simulink model "e03_MtrCtrl_MtrCtrl"  (R2024a)
settings: Solver=FixedStepDiscrete  StartTime=0.0  StopTime=1  FixedStep=mSim.dTime  MaxStep=Define.sModelSampleTime  RelTol=7.1420e-05
undefined symbols (not defined in the file): CnstCnst, CnstMde, CnstNr, E03CCTRL, E03INIT, E03LIM, E03MCMV, sTempGain
libraries: Lib_LPF x2
(part 2 of 3)

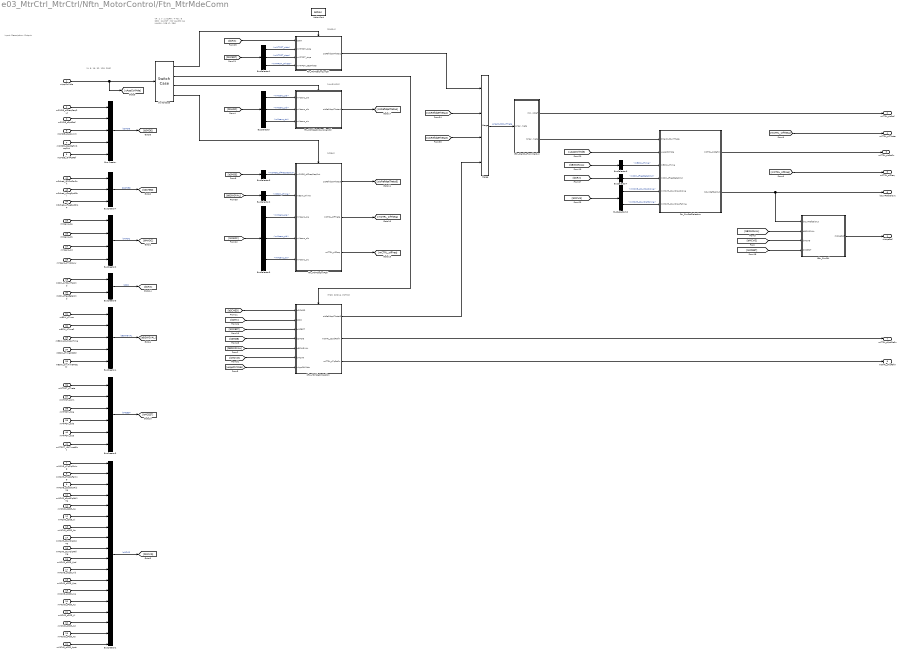
== system e03_MtrCtrl_MtrCtrl/Nftn_MotorControl/Ftn_MtrMdeComn ==
  note: [4, 8, 16, 32, 128, 256]
  note: Input:
      | Description:
      | Output:
  note: VF : 1
      | V : 2
      | CURR : 4
      | TQ : 8
      | SPD : 16
      | PST : 32
      | VALIGN: 64
      | IALIGN : 128
      | IF : 256
  note: [IF256]
  note: [CURR4]
  note: [IALIGN128]
  note: [TQ8, SPD16, PST32]
  uAppCtrlMde : Inport  Description=■ 설명: 모터 구동 제어 모드  OutMin=0  OutMax=32
      settings: AttributesFormatString=%<Description>
  mSMDE_sIfFreqSeqOut : Inport  Description=■ 설명: IF Control Frequency out  Port=2  OutMin=0  OutMax=54
      settings: AttributesFormatString=%<Description>
  mSMDE_sSpdRef : Inport  Description=■ 설명: Speed Reference  Port=3  OutMin=0  OutMax=11000
      settings: AttributesFormatString=%<Description>
  mSMDE_sSpdRefInSeqOut : Inport  Description=■ 설명: Speed Reference Slop Out  Port=4  OutMin=0  OutMax=11000
      settings: AttributesFormatString=%<Description>
  mSMDE_i64PstRef : Inport  Description=■ 설명: Position Reference  Port=5
      settings: AttributesFormatString=%<Description>
  mSMDE_sSpdLimit : Inport  Description='■ 설명: 속도 제한값  Port=6
      settings: AttributesFormatString=%<Description>
  mMCVG_sTqSlpRising : Inport  Description=■ 설명: 토크 제어 지령 가속 기울기  Port=7
      settings: AttributesFormatString=%<Description>
  mMCVG_sTqSlpFalling : Inport  Description=■ 설명: 토크 제어 지령 감속 기울기  Port=8
      settings: AttributesFormatString=%<Description>
  mMCVG_sSpdSlpRising : Inport  Description=■ 설명: Speed Slop Rising Gain  Port=9  OutMin=0  OutMax=3000
      settings: AttributesFormatString=%<Description>
  mMCVG_sSpdSlpFalling : Inport  Description=■ 설명: Speed Slop Falling Gain  Port=10  OutMin=0  OutMax=3000
      settings: AttributesFormatString=%<Description>
  mMCVG_sSCG_Kp : Inport  Description=■ 설명: Speed Gain Kp Gain  Port=11  OutMin=0  OutMax=10
      settings: AttributesFormatString=%<Description>
  mMCVG_sSCG_Ki : Inport  Description=■ 설명: Speed Gain Ki Gain  Port=12  OutMin=0  OutMax=10
      settings: AttributesFormatString=%<Description>
  mMCVG_sSCG_Ka : Inport  Description=■ 설명: Speed Gain Ka Gain  Port=13  OutMin=0  OutMax=100
      settings: AttributesFormatString=%<Description>
  mMCVG_sCurrSlpRising : Inport  Description=■ 설명: Current Rising Slop Gain  Port=14  OutMin=0  OutMax=5000
      settings: AttributesFormatString=%<Description>
  mMCVG_sCurrSlpFalling : Inport  Description=■ 설명: Current Falling Slop Gain  Port=15  OutMin=0  OutMax=5000
      settings: AttributesFormatString=%<Description>
  mMCVG_sCCG_Kpd : Inport  Description=■ d축 전류 제어 게인 Kp  Port=16  OutMin=0  OutMax=100
      settings: AttributesFormatString=%<Description>
  mMCVG_sCCG_Kid : Inport  Description=■ d축 전류 제어 게인 Ki  Port=17  OutMin=0  OutMax=100
      settings: AttributesFormatString=%<Description>
  mMCVG_sCCG_Kpq : Inport  Description=■ 설명: Current Gain Kp Gain  Port=18  OutMin=0  OutMax=100
      settings: AttributesFormatString=%<Description>
  mMCVG_sCCG_Kiq : Inport  Description=■ 설명: Current Gain Ki Gain  Port=19  OutMin=0  OutMax=100
      settings: AttributesFormatString=%<Description>
  mMCVG_sPCG_Kp : Inport  Description=■ 설명: 위치 제어 게인 Kp  Port=20
      settings: AttributesFormatString=%<Description>
  mMCVG_sPCG_Ki : Inport  Description=■ 설명: 위치 제어 게인 Ki  Port=21
      settings: AttributesFormatString=%<Description>
  mMCVG_sPCG_Kd : Inport  Description=■ 설명: 위치 제어 게인 Kd  Port=22
      settings: AttributesFormatString=%<Description>
  mMCVG_sPCG_Ka : Inport  Description=■ 설명: 위치 제어 게인 Ka  Port=23
      settings: AttributesFormatString=%<Description>
  mMCVG_sPCG_Apst : Inport  Description=■ 설명: 가속도 게인  Port=24
      settings: AttributesFormatString=%<Description>
  mMsens_sIa : Inport  Description=■ 설명: 모터 A상 전류  Port=25  OutMin=-162.6  OutMax=162.6
      settings: AttributesFormatString=%<Description>
  mMsens_sIb : Inport  Description=■ 설명: 모터 B상 전류  Port=26  OutMin=-162.6  OutMax=162.6
      settings: AttributesFormatString=%<Description>
  mMsens_sIc : Inport  Description=■ 설명: 모터 C상 전류  Port=27  OutMin=-325.2  OutMax=325.2
      settings: AttributesFormatString=%<Description>
  mMsens_sHVdcLow : Inport  Description=■ 설명: HVdc 전압  Port=28  OutMin=0  OutMax=1000
      settings: AttributesFormatString=%<Description>
  mCRX_sVltCurrTqCmd : Inport  Description=■ 설명: uVltCurrTqCmd(Voltage / Current / Torque Reference)  Port=29  OutMin=-398.3  OutMax=398.3
      settings: AttributesFormatString=%<Description>
  mCRX_sFreqBetaCmd : Inport  Description=■ 설명: uFreqBetaCmd(Frequency / Beta Reference)  Port=30  OutMin=0  OutMax=409.5
      settings: AttributesFormatString=%<Description>
  mBSW_sTime : Inport  Description=■ 설명: 주기, sTime (1/14kH)  Port=31  OutMin=0  OutMax=0.0000714286
      settings: AttributesFormatString=%<Description>
  mBSW_sTime2 : Inport  Description=■ 설명: sTime * 2  Port=32  OutMin=0  OutMax=0.000142857
      settings: AttributesFormatString=%<Description>
  mBSW_sOutloopTime : Inport  Description=■ 설명: sTime * 10  Port=33  OutMin=0  OutMax=0.000714286
      settings: AttributesFormatString=%<Description>
  mBSW_sTimePstCtrl : Inport  Description=■ 설명: Main Task 30배 주기  Port=34
      settings: AttributesFormatString=%<Description>
  mBSW_sInvTimePstCtrl : Inport  Description=■ 설명: mBSW_sTimePstCtrl의 역수  Port=35
      settings: AttributesFormatString=%<Description>
  mMTPST_sTheta : Inport  Description=■ 설명: Rotor Position  Port=36  OutMin=0  OutMax=6.2832
      settings: AttributesFormatString=%<Description>
  mMTPST_sWm : Inport  Description=■ 설명: 기계 각속도 (Wm = 12000 * 2pi/60)  Port=37  OutMin=0  OutMax=1256.63706
      settings: AttributesFormatString=%<Description>
  mMTPST_sWe : Inport  Description=■ 설명: 전기 각속도 (We = Wm * Poles)  Port=38  OutMin=0  OutMax=5026.55
      settings: AttributesFormatString=%<Description>
  mMTPST_sIde : Inport  Description=■ 설명: sIde  Port=39  OutMin=-398.3  OutMax=398.3
      settings: AttributesFormatString=%<Description>
  mMTPST_sIqe : Inport  Description=■ 설명: sIqe  Port=40  OutMin=-398.3  OutMax=398.3
      settings: AttributesFormatString=%<Description>
  mMTPST_i64TurretPst : Inport  Description=■ 설명: Turret Position  Port=41
      settings: AttributesFormatString=%<Description>
  mSched_i32CntForSch : Inport  Description=■ 설명: 메인 스케쥴 카운터  Port=42
      settings: AttributesFormatString=%<Description>
  mSched_uFlagSpdCtrl : Inport  Description=■ 설명: Speed Control 스케쥴 카운터  Port=43  OutMin=0  OutMax=1
      settings: AttributesFormatString=%<Description>
  mSched_uFlagSpdSlop : Inport  Description=■ 설명: 속도 지령 Slop 스케쥴 카운터  Port=44  OutMin=0  OutMax=1
      settings: AttributesFormatString=%<Description>
  ActionPort : ActionPort  ActionPortLabel=case [ 4 8 16 32 128 256 ]:
  Bus Creator : BusCreator  Inputs=5
  BusCreator1 : BusCreator  Inputs=18
  BusCreator2 : BusCreator  Inputs=4
  BusCreator3 : BusCreator  Inputs=2
  BusCreator4 : BusCreator  Inputs=5
  BusCreator5 : BusCreator  Inputs=6
  BusCreator7 : BusCreator  Inputs=3
  BusSelector : BusSelector  OutputSignals=mMsens_sIa,mMsens_sIb,mMsens_sIc
  BusSelector1 : BusSelector  OutputSignals=mMTPST_sIde,mMTPST_sIqe,mMTPST_sTheta
  BusSelector10 : BusSelector  OutputSignals=mMCVG_sCurrSlpRising,mMCVG_sCurrSlpFalling
  BusSelector2 : BusSelector  OutputSignals=mBSW_sTime
  BusSelector3 : BusSelector  OutputSignals=mSMDE_sIfFreqSeqOut
  BusSelector5 : BusSelector  OutputSignals=mMsens_sIa,mMsens_sIb,mMsens_sIc
  BusSelector6 : BusSelector  OutputSignals=mBSW_sTime
  BusSelector7 : BusSelector  OutputSignals=mCRX_sFreqBetaCmd
  Ftn_CurrRefSelection : Subsystem  TreatAsAtomicUnit=on
      settings: RTWSystemCode=Nonreusable function  RTWFcnNameOpts=Use subsystem name
  Ftn_MtrMdeCmCurrAlignCtrl : Subsystem
      settings: RTWSystemCode=Nonreusable function  RTWFcnNameOpts=Use subsystem name
  Ftn_MtrMdeCmCurrCtrl : Subsystem  Description=Current Control
      settings: RTWSystemCode=Nonreusable function  RTWFcnNameOpts=Use subsystem name
  Ftn_MtrMdeCmIFCtrl : Subsystem  Description=IF_Current
      settings: RTWSystemCode=Nonreusable function  RTWFcnNameOpts=Use subsystem name
  Merge : Merge  Inputs=4
  Nftn_CurrCtrl : Subsystem
      settings: RTWSystemCode=Nonreusable function  RTWFcnNameOpts=Use subsystem name
  Nftn_GenBusFromMerOut : Subsystem
  Nftn_MtrMdeCmSpdCm : Subsystem
      settings: RTWSystemCode=Inline  RTWFcnNameOpts=Use subsystem name
  SwitchCase : SwitchCase  CaseConditions={ 4, [8,16, 32], 128}
  sVdqeRef : Outport  Description=|  OutMin=-1000  OutMax=1000  VectorParamsAs1DForOutWhenUnconnected=off
      | ■ 설명: 전압 지령
      | -.[0] : d축 전압 지령
      | -.[1] : q축 전압 지령
      settings: AttributesFormatString=%<Description>
  mCTRL_sIsRef : Outport  Description=■ 설명: 전류 지령  Port=2  OutMin=-49.498  OutMax=49.498  VectorParamsAs1DForOutWhenUnconnected=off
      settings: AttributesFormatString=%<Description>
  mCTRL_sIsRefIn : Outport  Description=■ 설명: 전류 지령 (이전 값 / Unit Delay)  Port=3  OutMin=-49.498  OutMax=49.498  VectorParamsAs1DForOutWhenUnconnected=off
      settings: AttributesFormatString=%<Description>
  mCTRL_sIfTheta : Outport  Description=■ 설명: (IF 제어시) 추정 위치  Port=4  OutMin=0  OutMax=6.2832  VectorParamsAs1DForOutWhenUnconnected=off
      settings: AttributesFormatString=%<Description>
  mCTRL_sIfFreq : Outport  Description=■ 설명: (IF 제어시) 주파수 지령  Port=5  OutMin=0  OutMax=54  VectorParamsAs1DForOutWhenUnconnected=off
      settings: AttributesFormatString=%<Description>
  bCurrRefSelOut : Outport  Description=|  Port=6  VectorParamsAs1DForOutWhenUnconnected=off
      | ■ 설명: 제어 모드 전류 출력 Mux 신호
      | -.[0] : d축 전류 지령
      | -.[1] : q축 전류 지령
      | -.[2] : d축 전류
      | -.[3] : q축 전류
      | -.[4] : 추정 위치
      settings: AttributesFormatString=%<Description>
  mCTRL_sSpdRefIn : Outport  Description=■ 설명: Speed Reference  Port=7  OutMin=0  OutMax=11000  VectorParamsAs1DForOutWhenUnconnected=off
      settings: AttributesFormatString=%<Description>
  mCTRL_sTqRefIn : Outport  Description=■ 설명: Tq Slop Reference  Port=8  OutMin=1.5  OutMax=11.4  VectorParamsAs1DForOutWhenUnconnected=off
      settings: AttributesFormatString=%<Description>
  wires:
  [bBSWGVAL] -> Nftn_CurrCtrl/2(bBSWGVAL)
  Nftn_CurrCtrl/1(sVdqeRef) -> sVdqeRef/1
  SwitchCase/1 -> Ftn_MtrMdeCmCurrCtrl/Action
  uAppCtrlMde/1 -> SwitchCase/1, [uAppCtrlMde]
  Ftn_MtrMdeCmIFCtrl/3(mCTRL_sIfFreq) -> [mCTRL_sIfFreq]
  [bMCEST] -> Nftn_CurrCtrl/4(bMCEST)
  Ftn_CurrRefSelection/2(bCurrRefSelOut) -> bCurrRefSelOut/1, Nftn_CurrCtrl/1(bCurrRefSelOut)
  [uAppCtrlMde] -> Ftn_CurrRefSelection/2(uAppCtrlMde)
  SwitchCase/3 -> Ftn_MtrMdeCmCurrAlignCtrl/Action
  SwitchCase/4 -> Ftn_MtrMdeCmIFCtrl/Action
  Ftn_CurrRefSelection/1(mCTRL_sIsRefIn) -> mCTRL_sIsRefIn/1
  [mCTRL_sIfFreq] -> mCTRL_sIfFreq/1
  Ftn_MtrMdeCmIFCtrl/2(mCTRL_sIfTheta) -> [mCTRL_sIfTheta]
  [bMCVG] -> Nftn_CurrCtrl/3(bMCVG)
  Ftn_MtrMdeCmCurrCtrl/1(sIsRefIdqeTheta1) -> Merge/1
  Ftn_MtrMdeCmIFCtrl/1(sIsRefIdqeTheta3) -> [sIsRefIdqeTheta3]
  [sIsRefIdqeTheta3] -> Merge/3
  [sIsRefIdqeTheta4] -> Merge/2
  Ftn_MtrMdeCmCurrAlignCtrl/1(sIsRefIdqeTheta4) -> [sIsRefIdqeTheta4]
  Merge/1 -> Nftn_GenBusFromMerOut/1(aMerOutCCurrTheta)  "aMerOutCCurrTheta"
  Nftn_GenBusFromMerOut/1(mCTRL_sIsRef) -> mCTRL_sIsRef/1
  [mCTRL_sIfTheta] -> mCTRL_sIfTheta/1
  Nftn_MtrMdeCmSpdCm/1(sIsRefIdqeTheta5) -> Merge/4
  Nftn_MtrMdeCmSpdCm/2(mCTRL_sSpdRefIn) -> mCTRL_sSpdRefIn/1
  Nftn_MtrMdeCmSpdCm/3(mCTRL_sTqRefIn) -> mCTRL_sTqRefIn/1
  [bCRX] -> Nftn_MtrMdeCmSpdCm/2(bCRX)
  [bMCEST] -> Nftn_MtrMdeCmSpdCm/3(bMCEST)
  [bSMDE] -> Nftn_MtrMdeCmSpdCm/4(bSMDE)
  [bBSWGVAL] -> Nftn_MtrMdeCmSpdCm/5(bBSWGVAL)
  [bMCVG] -> Nftn_MtrMdeCmSpdCm/6(bMCVG)
  [uAppCtrlMde] -> Nftn_MtrMdeCmSpdCm/7(uAppCtrlMde)
  BusSelector1/3 -> Ftn_MtrMdeCmCurrCtrl/4(mMTPST_sEstTheta)  "<mMTPST_sTheta>"
  BusSelector1/2 -> Ftn_MtrMdeCmCurrCtrl/3(mMTPST_sIqe)  "<mMTPST_sIqe>"
  BusSelector1/1 -> Ftn_MtrMdeCmCurrCtrl/2(mMTPST_sIde)  "<mMTPST_sIde>"
  [bMCEST] -> BusSelector1/1
  [bMADC] -> BusSelector/1
  BusSelector/1 -> Ftn_MtrMdeCmCurrAlignCtrl/1(mMsens_sIa)  "<mMsens_sIa>"
  BusSelector/2 -> Ftn_MtrMdeCmCurrAlignCtrl/2(mMsens_sIb)  "<mMsens_sIb>"
  BusSelector/3 -> Ftn_MtrMdeCmCurrAlignCtrl/3(mMsens_sIc)  "<mMsens_sIc>"
  [bCRX] -> Ftn_MtrMdeCmCurrCtrl/1(bCRX)
  BusSelector3/1 -> Ftn_MtrMdeCmIFCtrl/1(mSMDE_sIfFreqSeqOut)  "<mSMDE_sIfFreqSeqOut>"
  [bSMDE] -> BusSelector3/1
  BusSelector2/1 -> Ftn_MtrMdeCmIFCtrl/2(mBSW_sTime)  "<mBSW_sTime>"
  [bBSWGVAL] -> BusSelector2/1
  BusSelector5/1 -> Ftn_MtrMdeCmIFCtrl/3(mMsens_sIa)  "<mMsens_sIa>"
  BusSelector5/2 -> Ftn_MtrMdeCmIFCtrl/4(mMsens_sIb)  "<mMsens_sIb>"
  BusSelector5/3 -> Ftn_MtrMdeCmIFCtrl/5(mMsens_sIc)  "<mMsens_sIc>"
  [bMADC] -> BusSelector5/1
  SwitchCase/2 -> Nftn_MtrMdeCmSpdCm/Action
  BusSelector6/1 -> Ftn_CurrRefSelection/3(mBSW_sTime)  "<mBSW_sTime>"
  [bBSWGVAL] -> BusSelector6/1
  BusSelector7/1 -> Ftn_CurrRefSelection/4(mCRX_sFreqBetaCmd)  "<mCRX_sFreqBetaCmd>"
  [bCRX] -> BusSelector7/1
  [bMCVG] -> BusSelector10/1
  BusSelector10/2 -> Ftn_CurrRefSelection/6(mMCVG_sCurrSlopFalling)  "<mMCVG_sCurrSlpFalling>"
  BusSelector10/1 -> Ftn_CurrRefSelection/5(mMCVG_sCurrSlopRising)  "<mMCVG_sCurrSlpRising>"
  Nftn_GenBusFromMerOut/2(bMerOutCurrTheta) -> Ftn_CurrRefSelection/1(bMerOutCurrTheta)
  mSMDE_sIfFreqSeqOut/1 -> Bus Creator/1
  mSMDE_sSpdRef/1 -> Bus Creator/2
  mSMDE_sSpdRefInSeqOut/1 -> Bus Creator/4
  Bus Creator/1 -> [bSMDE]  "bSMDE"
  mMCVG_sSpdSlpRising/1 -> BusCreator1/3
  mMCVG_sSpdSlpFalling/1 -> BusCreator1/4
  mMCVG_sSCG_Kp/1 -> BusCreator1/5
  mMCVG_sCCG_Kiq/1 -> BusCreator1/13
  mMCVG_sCCG_Kpq/1 -> BusCreator1/12
  mMCVG_sCurrSlpFalling/1 -> BusCreator1/9
  mMCVG_sCurrSlpRising/1 -> BusCreator1/8
  mMCVG_sSCG_Ka/1 -> BusCreator1/7
  mMCVG_sSCG_Ki/1 -> BusCreator1/6
  BusCreator1/1 -> [bMCVG]  "bMCVG"
  mMsens_sIa/1 -> BusCreator2/1
  BusCreator2/1 -> [bMADC]  "bMADC"
  mMsens_sIb/1 -> BusCreator2/2
  mMsens_sIc/1 -> BusCreator2/3
  mMsens_sHVdcLow/1 -> BusCreator2/4
  mCRX_sVltCurrTqCmd/1 -> BusCreator3/1
  mCRX_sFreqBetaCmd/1 -> BusCreator3/2
  BusCreator3/1 -> [bCRX]  "bCRX"
  mBSW_sTime/1 -> BusCreator4/1
  mBSW_sTime2/1 -> BusCreator4/2
  mBSW_sOutloopTime/1 -> BusCreator4/3
  BusCreator4/1 -> [bBSWGVAL]  "bBSWGVAL"
  mMTPST_sTheta/1 -> BusCreator5/1
  mMTPST_sWm/1 -> BusCreator5/2
  mMTPST_sWe/1 -> BusCreator5/3
  mMTPST_sIde/1 -> BusCreator5/4
  mMTPST_sIqe/1 -> BusCreator5/5
  BusCreator5/1 -> [bMCEST]  "bMCEST"
  mSched_uFlagSpdCtrl/1 -> BusCreator7/2
  mSched_uFlagSpdSlop/1 -> BusCreator7/3
  BusCreator7/1 -> [bSCHED]  "bSCHED"
  [bSCHED] -> Nftn_MtrMdeCmSpdCm/1(bSCHED)
  mMCVG_sCCG_Kpd/1 -> BusCreator1/10
  mMCVG_sCCG_Kid/1 -> BusCreator1/11
  mMCVG_sTqSlpRising/1 -> BusCreator1/1
  mMCVG_sTqSlpFalling/1 -> BusCreator1/2
  mMCVG_sPCG_Kp/1 -> BusCreator1/14
  mMCVG_sPCG_Ki/1 -> BusCreator1/15
  mMCVG_sPCG_Kd/1 -> BusCreator1/16
  mMCVG_sPCG_Ka/1 -> BusCreator1/17
  mMCVG_sPCG_Apst/1 -> BusCreator1/18
  mBSW_sTimePstCtrl/1 -> BusCreator4/4
  mSched_i32CntForSch/1 -> BusCreator7/1
  mSMDE_i64PstRef/1 -> Bus Creator/5
  mMTPST_i64TurretPst/1 -> BusCreator5/6
  mBSW_sInvTimePstCtrl/1 -> BusCreator4/5
  mSMDE_sSpdLimit/1 -> Bus Creator/3

== system e03_MtrCtrl_MtrCtrl/Nftn_MotorControl/Ftn_SelectionCtrlMde ==
  note: Input:
      | Description:
      | Output:
  mDIAG_uFltStat : Inport  Description=■ 설명: 진단 상태  OutMin=0  OutMax=1
      settings: AttributesFormatString=%<Description>
  mSMDE_uFlagInverterOut : Inport  Description=■ 설명: FlagInverter Out  Port=2  OutMin=0  OutMax=1
      settings: AttributesFormatString=%<Description>
  mSMDE_uMtrCtrlMde : Inport  Description=■ 설명: 모터 제어 모드(Motor Control Mode)  Port=3  OutMin=0  OutMax=32
      settings: AttributesFormatString=%<Description>
  CB_u16True : Constant  OutDataTypeStr=uint16
  CB_u16Zero : Constant  Value=0  OutDataTypeStr=uint16
  Chart : Stateflow chart
      settings: RTWSystemCode=Nonreusable function  RTWFcnNameOpts=Use subsystem name  PortSchema="{\"entries\":[{\"content\":{\"sides\":[{\"content\":{\"connectorIds\":[\"In2\",\"In1\",\"In3\",\"In4\",\"In5\"]},\"type\":\"ConnectorPlacement.EquallySpacedRectSide\",\"uuid\":\"2d3631c7-4ca5-451f-a483-2145aabb85be\"},{\"content\":{\"connectorIds\":[\"Out1\"],\"side\":\"RIGHT\"},\"type\":\"ConnectorPlacement.EquallySpacedRectSide\",\"uuid\":\"88d0d170-d09d-4d9e-b71c-3199afb1d184\"},{\"content\":{\"side\":\"TOP\"},\"type\":\"ConnectorPlacement.EquallySpacedRectSide\",\"uuid\":\"83cc8dd3-cda1-47f0-aa67-0691b9a18feb\"}]},\"type\":\"ConnectorPlacement.EquallySpacedConnector\",\"uuid\":\"609d7b9c-ebea-4372-949b-9312fe794362\"}],\"packageUris\":[\"http://schema.mathworks.com/mf0/Connector/R2020b\"],\"version\":\"1.0\"}"
  uAppCtrlMde : Outport  Description=■ 설명: 모터 구동 제어 모드  OutMin=0  OutMax=32
      settings: AttributesFormatString=%<Description>
  wires:
  Chart/1(uAppCtrlMde) -> uAppCtrlMde/1
  mSMDE_uFlagInverterOut/1 -> Chart/2(mSMDE_uFlagInverterOut)
  mSMDE_uMtrCtrlMde/1 -> Chart/1(mSMDE_uMtrCtrlMde)
  CB_u16Zero/1 -> Chart/4(u16Zero)  "u16Zero"
  CB_u16True/1 -> Chart/5(u16True)  "u16True"
  mDIAG_uFltStat/1 -> Chart/3(mDIAG_uFltStat)

== system e03_MtrCtrl_MtrCtrl/Nftn_MotorControl/Nftn_MerVC ==
  note: Input:
      | Description:
      | Output:
  aMerVC : Inport
  Demux : Demux  Outputs=3
  SignalConversion : SignalConversion  OverrideOpt=off
  SignalConversion1 : SignalConversion  OverrideOpt=off
  SignalConversion2 : SignalConversion  OverrideOpt=off
  mCTRL_sThetaCtrl : Outport
  mCTRL_sVdeRef : Outport  Port=2
  mCTRL_sVqeRef : Outport  Port=3
  wires:
  aMerVC/1 -> Demux/1
  SignalConversion/1 -> mCTRL_sVdeRef/1  "mCTRL_sVdeRef"
  Demux/2 -> SignalConversion1/1  "MerOut_sVqeRef"
  Demux/1 -> SignalConversion/1  "MerOut_sVdeRef"
  SignalConversion2/1 -> mCTRL_sThetaCtrl/1  "mCTRL_sThetaCtrl"
  SignalConversion1/1 -> mCTRL_sVqeRef/1  "mCTRL_sVqeRef"
  Demux/3 -> SignalConversion2/1  "MerOut_sThetaCtrl"

== system e03_MtrCtrl_MtrCtrl/Nftn_MotorControl/Ftn_MtrCtrlMdeVCtrl/Ftn_VCtrlSlop ==
  note: Input:
      | Description:
      | Output:
  mCRX_sVltCurrTqCmd : Inport  Description=■ 설명: uVltCurrTqCmd(Voltage / Current / Torque Reference)  OutMin=-398.3  OutMax=398.3
      settings: AttributesFormatString=%<Description>
  mBSW_sTime : Inport  Description=■ 설명: 주기, sTime (1/10kh)  Port=2  OutMin=0  OutMax=0.0000714286
      settings: AttributesFormatString=%<Description>
  CB_E03MCMV_sVltSlopFalling : Constant  Value=E03MCMV.sVltSlopFalling
  CB_E03MCMV_sVltSlopRising : Constant  Value=E03MCMV.sVltSlopRising
  Product : Product
  Product1 : Product
  RelationalOperator1 : RelationalOperator  Operator=<  InputSameDT=off
  RelationalOperator2 : RelationalOperator  Operator=>  InputSameDT=off
  Sum : Sum
  Sum1 : Sum  Inputs=+-
  Switch1 : Switch  Criteria=u2 ~= 0  SaturateOnIntegerOverflow=off  InputSameDT=off
  Switch2 : Switch  Criteria=u2 ~= 0  SaturateOnIntegerOverflow=off  InputSameDT=off
  UnitDelay1 : UnitDelay  InitialCondition=E03INIT.sVVltSlopVqeRefZ  SampleTime=-1  StateName=sVqeRefZ_V  HasFrameUpgradeWarning=on
      settings: AttributesFormatString=%<InitialCondition>
  sVVqeRef : Outport  Description=■ 설명: (V 제어 시) Vqe Reference  OutMin=-1000  OutMax=1000  VectorParamsAs1DForOutWhenUnconnected=off
      settings: AttributesFormatString=%<Description>
  wires:
  mBSW_sTime/1 -> Product1/1, Product/2
  Sum/1 -> Switch1/3, RelationalOperator1/2  "sBaudMax1V"
  Product/1 -> Sum/1  "sStepRisingV"
  Product1/1 -> Sum1/2  "sStepFallingV"
  RelationalOperator2/1 -> Switch2/2  "sTempVCtrl2"
  RelationalOperator1/1 -> Switch1/2  "sTempVCtrl1"
  Sum1/1 -> RelationalOperator2/2, Switch2/3  "sBaudMinV"
  [sVVqeRefZ] -> Sum1/1, Sum/2
  Switch1/1 -> RelationalOperator2/1, Switch2/1  "sBudMax2V"
  CB_E03MCMV_sVltSlopFalling/1 -> Product1/2  "sVltSlopsFalling"
  CB_E03MCMV_sVltSlopRising/1 -> Product/1  "sVltSlopRising"
  Switch2/1 -> sVVqeRef/1, UnitDelay1/1  "sVVqeRef"
  UnitDelay1/1 -> [sVVqeRefZ]  "sVVqeRefZ"
  mCRX_sVltCurrTqCmd/1 -> RelationalOperator1/1, Switch1/1

== system e03_MtrCtrl_MtrCtrl/Nftn_MotorControl/Ftn_MtrCtrlMdeVCtrl/Nftn_MuxVCtrl ==
  note: Input:
      | Description:
      | Output:
  sVqeRef_V : Inport  Description=■ 설명: (V/F제어 시) Vqe Reference  OutMin=-1000  OutMax=1000
      settings: AttributesFormatString=%<Description>
  mMTPST_sTheta : Inport  Description=■ 설명: Rotor Position  Port=2  OutMin=0  OutMax=6.2832
      settings: AttributesFormatString=%<Description>
  CB_sVdeRef : Constant  Value=0  OutDataTypeStr=single
  Mux1 : Mux  Inputs=3
  sVdqeRefTheta2 : Outport  Description=|  OutMin=-1000  OutMax=1000
      | ■ 설명: 제어 모드 전류 출력 Mux 신호
      | -.[0] : d축 전압 지령
      | -.[1] : q축 전압 지령
      | -.[2] : Theta control cmd
      settings: AttributesFormatString=%<Description>
  wires:
  Mux1/1 -> sVdqeRefTheta2/1  "sVdqeRefTheta2"
  CB_sVdeRef/1 -> Mux1/1  "sVdeRef"
  sVqeRef_V/1 -> Mux1/2
  mMTPST_sTheta/1 -> Mux1/3

== system e03_MtrCtrl_MtrCtrl/Nftn_MotorControl/Ftn_MtrCtrlMdeVFCtrl/Ftn_VfCtrlSlop ==
  note: Input:
      | Description:
      | Output:
  mCRX_sVltCurrTqCmd : Inport  Description=■ 설명: uVltCurrTqCmd(Voltage / Current / Torque Reference)  OutMin=-398.3  OutMax=398.3
      settings: AttributesFormatString=%<Description>
  mBSW_sTime : Inport  Description=■ 설명: 주기, sTime (1/10kh)  Port=2  OutMin=0  OutMax=0.0000714286
      settings: AttributesFormatString=%<Description>
  CB_E03MCMV_sVltSlopFalling : Constant  Value=E03MCMV.sVltSlopFalling
  CB_E03MCMV_sVltSlopRising : Constant  Value=E03MCMV.sVltSlopRising
  Product : Product
  Product1 : Product
  RelationalOperator1 : RelationalOperator  Operator=<  InputSameDT=off
  RelationalOperator2 : RelationalOperator  Operator=>  InputSameDT=off
  Sum : Sum
  Sum1 : Sum  Inputs=+-
  Switch1 : Switch  Criteria=u2 ~= 0  SaturateOnIntegerOverflow=off  InputSameDT=off
  Switch2 : Switch  Criteria=u2 ~= 0  SaturateOnIntegerOverflow=off  InputSameDT=off
  UnitDelay1 : UnitDelay  InitialCondition=E03INIT.sVfVltSlopVqeRefZ  SampleTime=-1  StateName=sVqeRefZ_VF  HasFrameUpgradeWarning=on
      settings: AttributesFormatString=%<InitialCondition>
  sVfVqeRef : Outport  Description=■ 설명: (V/F제어 시) Vqe Reference  OutMin=-1000  OutMax=1000  VectorParamsAs1DForOutWhenUnconnected=off
      settings: AttributesFormatString=%<Description>
  wires:
  mBSW_sTime/1 -> Product/2, Product1/1
  Sum/1 -> RelationalOperator1/2, Switch1/3  "sBaudMax1VF"
  Product/1 -> Sum/1  "sStepRisingVF"
  Product1/1 -> Sum1/2  "sStepFallingVF"
  RelationalOperator2/1 -> Switch2/2  "sTempVFCtrl2"
  RelationalOperator1/1 -> Switch1/2  "sTempVFCtrl1"
  Sum1/1 -> Switch2/3, RelationalOperator2/2  "sBaudMinVF"
  [sVfVqeRefZ] -> Sum/2, Sum1/1
  Switch1/1 -> RelationalOperator2/1, Switch2/1  "sBudMax2VF"
  CB_E03MCMV_sVltSlopFalling/1 -> Product1/2  "sVltSlopsFalling"
  CB_E03MCMV_sVltSlopRising/1 -> Product/1  "sVltSlopRising"
  mCRX_sVltCurrTqCmd/1 -> RelationalOperator1/1, Switch1/1
  Switch2/1 -> sVfVqeRef/1, UnitDelay1/1  "sVfVqeRef"
  UnitDelay1/1 -> [sVfVqeRefZ]  "sVfVqeRefZ"

== system e03_MtrCtrl_MtrCtrl/Nftn_MotorControl/Ftn_MtrCtrlMdeVFCtrl/Nftn_MuxVFCtrl ==
  note: Input:
      | Description:
      | Output:
  mCRX_sFreqBetaCmd : Inport  Description=■ 설명: uFreqBetaCmd(Frequency / Beta Reference)  OutMin=0  OutMax=409.5
      settings: AttributesFormatString=%<Description>
  sVfVqeRef : Inport  Description=■ 설명: (V/F제어 시) Vqe Reference  Port=2  OutMin=-1000  OutMax=1000
      settings: AttributesFormatString=%<Description>
  mBSW_sTime : Inport  Description=■ 설명: 주기, sTime (1/10kh)  Port=3  OutMin=0  OutMax=0.0000714286
      settings: AttributesFormatString=%<Description>
  CB_C_PI2 : Constant  Value=CnstCnst.C_PI2
  CB_sVdeRef : Constant  Value=0  OutDataTypeStr=single
  Chart_MtrCtrlMdeVFCtrl : Stateflow chart
      settings: RTWSystemCode=Nonreusable function  RTWFcnNameOpts=Use subsystem name
  Mux1 : Mux  Inputs=3
  sVdqeRefTheta1 : Outport  Description=|  OutMin=-1000  OutMax=1000
      | ■ 설명: 제어 모드 전류 출력 Mux 신호
      | -.[0] : d축 전압 지령
      | -.[1] : q축 전압 지령
      | -.[2] : Theta control cmd
      settings: AttributesFormatString=%<Description>
  wires:
  mBSW_sTime/1 -> Chart_MtrCtrlMdeVFCtrl/2(mBSW_sTime)
  Chart_MtrCtrlMdeVFCtrl/1(sVfThetaRef) -> Mux1/3
  sVfVqeRef/1 -> Mux1/2
  CB_sVdeRef/1 -> Mux1/1  "sVdeRef"
  Mux1/1 -> sVdqeRefTheta1/1  "sVdqeRefTheta1"
  mCRX_sFreqBetaCmd/1 -> Chart_MtrCtrlMdeVFCtrl/1(mCRX_sFreqBetaCmd)
  CB_C_PI2/1 -> Chart_MtrCtrlMdeVFCtrl/3(C_PI2)  "C_PI2"

== system e03_MtrCtrl_MtrCtrl/Nftn_MotorControl/Ftn_MtrMdeComn/Ftn_CurrRefSelection ==
  note: Input:
      | Description:
      | Output:
  bMerOutCurrTheta : Inport  Description=|
      | ■ 설명: 제어 모드 전류 출력 Mux 신호
      | -.[0] : 전압/전류/토크 지령, [1] : d축 전류
      | -.[2] : q축 전류, [3] : 추정 위치
      settings: AttributesFormatString=%<Description>
  uAppCtrlMde : Inport  Description=■ 설명: 모터 구동 제어 모드  Port=2  OutMin=0  OutMax=32
      settings: AttributesFormatString=%<Description>
  mBSW_sTime : Inport  Description=■ 설명: 주기, sTime (1/14kH)  Port=3  OutMin=0  OutMax=0.0000714286
      settings: AttributesFormatString=%<Description>
  mCRX_sFreqBetaCmd : Inport  Description=■ 설명: uFreqBetaCmd(Frequency / Beta Reference)  Port=4  OutMin=0  OutMax=409.5
      settings: AttributesFormatString=%<Description>
  mMCVG_sCurrSlopRising : Inport  Description=■ 설명: Current Rising Slop Gain  Port=5  OutMin=0  OutMax=5000
      settings: AttributesFormatString=%<Description>
  mMCVG_sCurrSlopFalling : Inport  Description=■ 설명: Current Falling Slop Gain  Port=6  OutMin=0  OutMax=5000
      settings: AttributesFormatString=%<Description>
  BusSelector : BusSelector  OutputSignals=mCTRL_sIsRef,sIde,sIqe,sAppTheta
  Nftn_GenArryOut : Subsystem
  Nftn_SftCurrMde : Subsystem
      settings: RTWSystemCode=Nonreusable function  RTWFcnNameOpts=Use subsystem name
  mCTRL_sIsRefIn : Outport  Description=■ 설명: 전류 지령 (이전 값 / Unit Delay)  OutMin=-398.3  OutMax=398.3  VectorParamsAs1DForOutWhenUnconnected=off
      settings: AttributesFormatString=%<Description>
  bCurrRefSelOut : Outport  Description=|  Port=2
      | ■ 설명: 제어 모드 전류 출력 Mux 신호
      | -.[0] : d축 전류 지령
      | -.[1] : q축 전류 지령
      | -.[2] : d축 전류
      | -.[3] : q축 전류
      | -.[4] : 추정 위치
      settings: AttributesFormatString=%<Description>
  wires:
  uAppCtrlMde/1 -> Nftn_SftCurrMde/1(uAppCtrlMde)
  Nftn_SftCurrMde/1(mCTRL_sIsRefIn) -> mCTRL_sIsRefIn/1
  Nftn_GenArryOut/1(bCurrRefSelOut) -> bCurrRefSelOut/1
  mBSW_sTime/1 -> Nftn_SftCurrMde/2(mBSW_sTime)
  mCRX_sFreqBetaCmd/1 -> Nftn_SftCurrMde/3(mCRX_sFreqBetaCmd)
  mMCVG_sCurrSlopRising/1 -> Nftn_SftCurrMde/4(mMCVG_sCurrSlopRising)
  mMCVG_sCurrSlopFalling/1 -> Nftn_SftCurrMde/5(mMCVG_sCurrSlopFalling)
  bMerOutCurrTheta/1 -> BusSelector/1
  BusSelector/3 -> Nftn_GenArryOut/3(sIqe)  "<sIqe>"
  BusSelector/4 -> Nftn_GenArryOut/4(sAppTheta)  "<sAppTheta>"
  BusSelector/2 -> Nftn_GenArryOut/2(sIde)  "<sIde>"
  BusSelector/1 -> Nftn_SftCurrMde/6(mCTRL_sIsRef)  "<mCTRL_sIsRef>"
  Nftn_SftCurrMde/2(sIdqeRef) -> Nftn_GenArryOut/1(sIdqeRef)

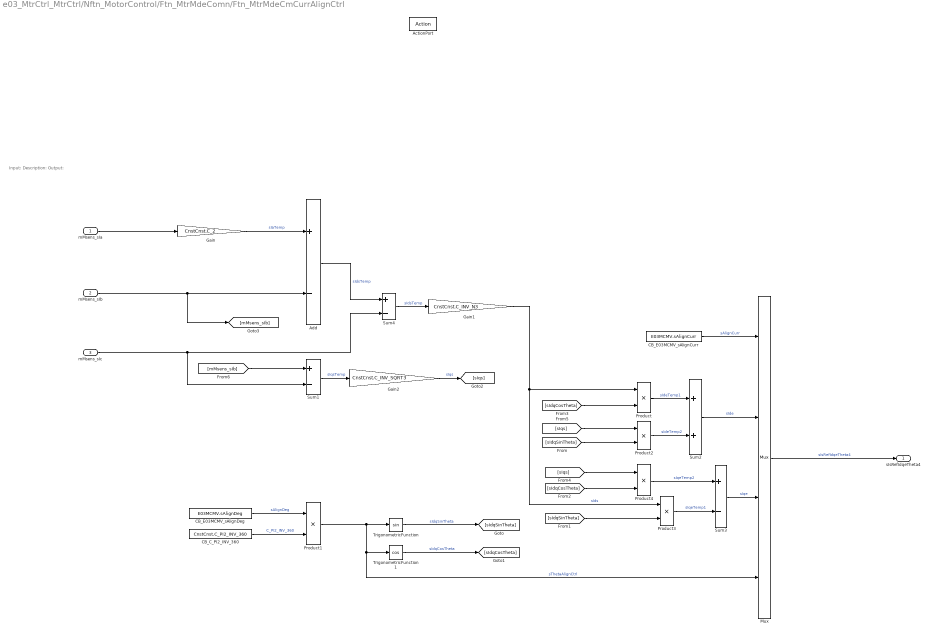
== system e03_MtrCtrl_MtrCtrl/Nftn_MotorControl/Ftn_MtrMdeComn/Ftn_MtrMdeCmCurrAlignCtrl ==
  note: Input:
      | Description:
      | Output:
  mMsens_sIa : Inport  Description=■ 설명: 모터 A상 전류  OutMin=-162.6  OutMax=162.6
      settings: AttributesFormatString=%<Description>
  mMsens_sIb : Inport  Description=■ 설명: 모터 B상 전류  Port=2  OutMin=-162.6  OutMax=162.6
      settings: AttributesFormatString=%<Description>
  mMsens_sIc : Inport  Description=■ 설명: 모터 B상 전류  Port=3  OutMin=-325.2  OutMax=325.2
      settings: AttributesFormatString=%<Description>
  ActionPort : ActionPort  ActionPortLabel=case [ 128 ]:
  Add : Sum  Inputs=+-
  CB_C_PI2_INV_360 : Constant  Value=CnstCnst.C_PI2_INV_360
  CB_E03MCMV_sAlignCurr : Constant  Value=E03MCMV.sAlignCurr
  CB_E03MCMV_sAlignDeg : Constant  Value=E03MCMV.sAlignDeg
  Gain : Gain  Gain=CnstCnst.C_2
  Gain1 : Gain  Gain=CnstCnst.C_INV_N3
  Gain2 : Gain  Gain=CnstCnst.C_INV_SQRT3
  Mux : Mux
  Product{,2..4} (4 alike) : Product  RndMeth=Zero
  Product1 : Product
  Sum1 : Sum  Inputs=+-
  Sum2 : Sum
  Sum3 : Sum  Inputs=+-
  Sum4 : Sum  Inputs=+-
  TrigonometricFunction : Trigonometry
  TrigonometricFunction1 : Trigonometry  Operator=cos
  sIsRefIdqeTheta4 : Outport  Description=|  OutMin=-398.3  OutMax=398.3
      | ■ 설명: 제어 모드 전류 출력 Mux 신호
      | -.[0] : 전압/전류/토크 지령
      | -.[1] : d축 전류
      | -.[2] : q축 전류
      | -.[3] : 추정 위치
      settings: AttributesFormatString=%<Description>
  wires:
  CB_E03MCMV_sAlignCurr/1 -> Mux/1  "sAlignCurr"
  CB_E03MCMV_sAlignDeg/1 -> Product1/1  "sAlignDeg"
  CB_C_PI2_INV_360/1 -> Product1/2  "C_PI2_INV_360"
  Product1/1 -> Mux/4, TrigonometricFunction1/1, TrigonometricFunction/1  "sThetaAlignCtrl"
  Sum4/1 -> Gain1/1  "sIdsTemp"
  Product4/1 -> Sum3/1  "sIqeTemp2"
  Gain/1 -> Add/1  "sIaTemp"
  [mMsens_sIb] -> Sum1/1
  Add/1 -> Sum4/1  "sIdsTemp"
  Gain2/1 -> [sIqs]  "sIqs"
  [sIdqCosTheta] -> Product4/2
  TrigonometricFunction1/1 -> [sIdqCosTheta]  "sIdqCosTheta"
  [sIqs] -> Product4/1
  [sIdqSinTheta] -> Product3/2
  [sIdqSinTheta] -> Product2/2
  mMsens_sIa/1 -> Gain/1
  TrigonometricFunction/1 -> [sIdqSinTheta]  "sIdqSinTheta"
  [sIqs] -> Product2/1
  Gain1/1 -> Product3/1, Product/1  "sIds"
  Product2/1 -> Sum2/2  "sIdeTemp2"
  [sIdqCosTheta] -> Product/2
  Product3/1 -> Sum3/2  "sIqeTemp1"
  Sum3/1 -> Mux/3  "sIqe"
  Sum1/1 -> Gain2/1  "sIqsTemp"
  Sum2/1 -> Mux/2  "sIde"
  mMsens_sIc/1 -> Sum1/2, Sum4/2
  mMsens_sIb/1 -> [mMsens_sIb], Add/2
  Product/1 -> Sum2/1  "sIdeTemp1"
  Mux/1 -> sIsRefIdqeTheta4/1  "sIsRefIdqeTheta4"

== system e03_MtrCtrl_MtrCtrl/Nftn_MotorControl/Ftn_MtrMdeComn/Ftn_MtrMdeCmCurrCtrl ==
  note: Input:
      | Description:
      | Output:
  bCRX : Inport  Description=■ 설명: uVltCurrTqCmd(Voltage / Current / Torque Reference)
      settings: AttributesFormatString=%<Description>
  mMTPST_sIde : Inport  Description=■ 설명: sIde  Port=2
      settings: AttributesFormatString=%<Description>
  mMTPST_sIqe : Inport  Description=■ 설명: sIqe  Port=3  OutMin=-398.3  OutMax=398.3
      settings: AttributesFormatString=%<Description>
  mMTPST_sEstTheta : Inport  Description=■ 설명: Rotor Position  Port=4  OutMin=0  OutMax=6.2832
      settings: AttributesFormatString=%<Description>
  ActionPort : ActionPort  ActionPortLabel=case [ 4 ]:
  BusSelector : BusSelector  OutputSignals=mCRX_sVltCurrTqCmd
  Mux : Mux
  sIsRefIdqeTheta1 : Outport  Description=|  OutMin=-398.3  OutMax=398.3  VectorParamsAs1DForOutWhenUnconnected=off
      | ■ 설명: 제어 모드 전류 출력 Mux 신호
      | -.[0] : 전압/전류/토크 지령
      | -.[1] : d축 전류
      | -.[2] : q축 전류
      | -.[3] : 추정 위치
      settings: AttributesFormatString=%<Description>
  wires:
  Mux/1 -> sIsRefIdqeTheta1/1  "sIsRefIdqeTheta1"
  mMTPST_sIde/1 -> Mux/2
  mMTPST_sEstTheta/1 -> Mux/4
  mMTPST_sIqe/1 -> Mux/3
  BusSelector/1 -> Mux/1  "<mCRX_sVltCurrTqCmd>"
  bCRX/1 -> BusSelector/1

== system e03_MtrCtrl_MtrCtrl/Nftn_MotorControl/Ftn_MtrMdeComn/Ftn_MtrMdeCmIFCtrl ==
  note: Input:
      | Description:
      | Output:
  note: VF : 1
      | V : 2
      | CURR : 4
      | TQ : 8
      | SPD : 16
      | PST : 32
      | VALIGN: 64
      | IALIGN : 128
      | IF : 256
  note: [TQ8, SPD 16 , PST32, IF256]
  mSMDE_sIfFreqSeqOut : Inport  Description=■ 설명: IF Control Frequency out  OutMin=0  OutMax=54
      settings: AttributesFormatString=%<Description>
  mBSW_sTime : Inport  Description=■ 설명: 주기, sTime (1/14kH)  Port=2  OutMin=0  OutMax=0.0000714286
      settings: AttributesFormatString=%<Description>
  mMsens_sIa : Inport  Description=■ 설명: 모터 A상 전류  Port=3  OutMin=-162.6  OutMax=162.6
      settings: AttributesFormatString=%<Description>
  mMsens_sIb : Inport  Description=■ 설명: 모터 B상 전류  Port=4  OutMin=-162.6  OutMax=162.6
      settings: AttributesFormatString=%<Description>
  mMsens_sIc : Inport  Description=■ 설명: 모터 C상 전류  Port=5  OutMin=-325.2  OutMax=325.2
      settings: AttributesFormatString=%<Description>
  ActionPort : ActionPort  ActionPortLabel=default:
  Ftn_MtrMdeCmIFCtrlB : Subsystem  TreatAsAtomicUnit=on
      settings: RTWSystemCode=Nonreusable function  RTWFcnNameOpts=Use subsystem name
  Nftn_MtrMdeCmIFCtrlA : Subsystem
      settings: RTWSystemCode=Nonreusable function  RTWFcnNameOpts=Use subsystem name
  sIsRefIdqeTheta3 : Outport  Description=|  OutMin=-398.3  OutMax=398.3  VectorParamsAs1DForOutWhenUnconnected=off
      | ■ 설명: 제어 모드 전류 출력 Mux 신호
      | -.[0] : 전압/전류/토크 지령
      | -.[1] : d축 전류
      | -.[2] : q축 전류
      | -.[3] : 추정 위치
      settings: AttributesFormatString=%<Description>
  mCTRL_sIfTheta : Outport  Description=■ 설명: (IF 제어시) 추정 위치  Port=2  OutMin=0  OutMax=6.2832
      settings: AttributesFormatString=%<Description>
  mCTRL_sIfFreq : Outport  Description=■ 설명: (IF 제어시) 주파수 지령  Port=3  OutMin=0  OutMax=54  VectorParamsAs1DForOutWhenUnconnected=off
      settings: AttributesFormatString=%<Description>
  wires:
  Nftn_MtrMdeCmIFCtrlA/1(mCTRL_sIfFreq) -> mCTRL_sIfFreq/1
  Nftn_MtrMdeCmIFCtrlA/2(mCTRL_sIfTheta) -> Ftn_MtrMdeCmIFCtrlB/1(mCTRL_sIfTheta), mCTRL_sIfTheta/1
  Nftn_MtrMdeCmIFCtrlA/3(sIfCurr) -> Ftn_MtrMdeCmIFCtrlB/2(sIfCurr)
  Ftn_MtrMdeCmIFCtrlB/1(sIsRefIdqeTheta3) -> sIsRefIdqeTheta3/1
  mMsens_sIa/1 -> Ftn_MtrMdeCmIFCtrlB/3(mMsens_sIa)
  mMsens_sIb/1 -> Ftn_MtrMdeCmIFCtrlB/4(mMsens_sIb)
  mMsens_sIc/1 -> Ftn_MtrMdeCmIFCtrlB/5(mMsens_sIc)
  mSMDE_sIfFreqSeqOut/1 -> Nftn_MtrMdeCmIFCtrlA/2(mSMDE_sIfFreqSeqOut)
  mBSW_sTime/1 -> Nftn_MtrMdeCmIFCtrlA/1(mBSW_sTime)

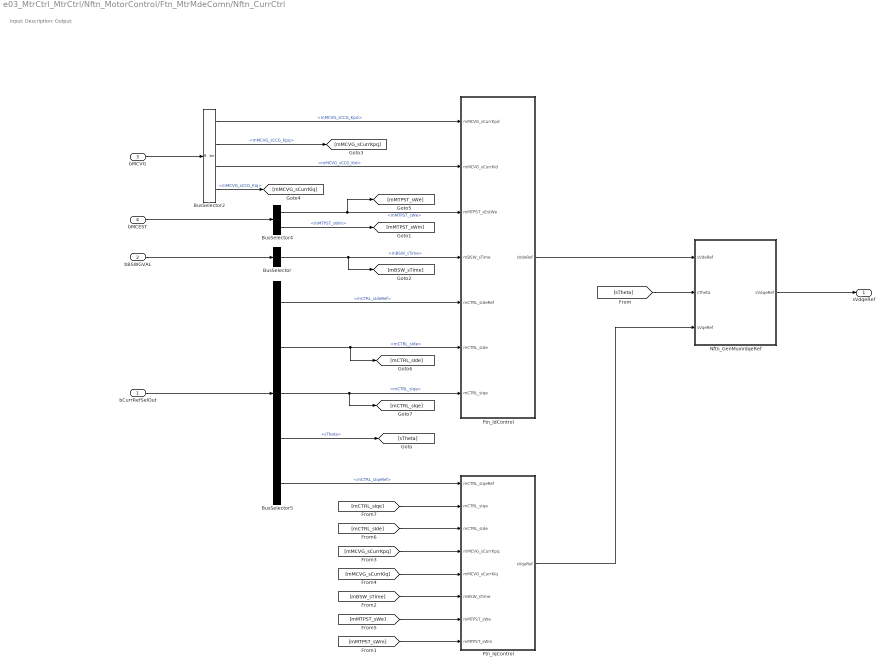
== system e03_MtrCtrl_MtrCtrl/Nftn_MotorControl/Ftn_MtrMdeComn/Nftn_CurrCtrl ==
  note: Input:
      | Description:
      | Output:
  bCurrRefSelOut : Inport
  bBSWGVAL : Inport  Port=2
  bMCVG : Inport  Port=3
  bMCEST : Inport  Port=4
  BusSelector : BusSelector  OutputSignals=mBSW_sTime
  BusSelector2 : BusSelector  OutputSignals=mMCVG_sCCG_Kpd,mMCVG_sCCG_Kpq,mMCVG_sCCG_Kid,mMCVG_sCCG_Kiq
  BusSelector4 : BusSelector  OutputSignals=mMTPST_sWe,mMTPST_sWm
  BusSelector5 : BusSelector  OutputSignals=mCTRL_sIdeRef,mCTRL_sIde,mCTRL_sIqe,sTheta,mCTRL_sIqeRef
  Ftn_IdControl : Subsystem  Description="/*  d-Axis Current Control  */"  Priority=1  TreatAsAtomicUnit=on
      settings: RTWSystemCode=Nonreusable function  RTWFcnNameOpts=Use subsystem name
  Ftn_IqControl : Subsystem  Description="/*  q-Axis Current Control  */"  Priority=2  TreatAsAtomicUnit=on
      settings: RTWSystemCode=Nonreusable function  RTWFcnNameOpts=Use subsystem name
  Nftn_GenMuxVdqeRef : Subsystem
  sVdqeRef : Outport  Description=■ Vdq 전압 지령  VectorParamsAs1DForOutWhenUnconnected=off
  wires:
  BusSelector/1 -> Ftn_IdControl/4(mBSW_sTime), [mBSW_sTime]  "<mBSW_sTime>"
  [mBSW_sTime] -> Ftn_IqControl/6(mBSW_sTime)
  bBSWGVAL/1 -> BusSelector/1
  Ftn_IdControl/1(sVdeRef) -> Nftn_GenMuxVdqeRef/1(sVdeRef)
  Ftn_IqControl/1(sVqeRef) -> Nftn_GenMuxVdqeRef/3(sVqeRef)
  Nftn_GenMuxVdqeRef/1(sVdqeRef) -> sVdqeRef/1
  [sTheta] -> Nftn_GenMuxVdqeRef/2(sTheta)
  bMCVG/1 -> BusSelector2/1
  BusSelector2/3 -> Ftn_IdControl/2(mMCVG_sCurrKid)  "<mMCVG_sCCG_Kid>"
  BusSelector2/1 -> Ftn_IdControl/1(mMCVG_sCurrKpd)  "<mMCVG_sCCG_Kpd>"
  [mMCVG_sCurrKpq] -> Ftn_IqControl/4(mMCVG_sCurrKpq)
  [mMCVG_sCurrKiq] -> Ftn_IqControl/5(mMCVG_sCurrKiq)
  bMCEST/1 -> BusSelector4/1
  BusSelector4/2 -> [mMTPST_sWm]  "<mMTPST_sWm>"
  BusSelector4/1 -> Ftn_IdControl/3(mMTPST_sEstWe), [mMTPST_sWe]  "<mMTPST_sWe>"
  [mMTPST_sWe] -> Ftn_IqControl/7(mMTPST_sWe)
  [mMTPST_sWm] -> Ftn_IqControl/8(mMTPST_sWm)
  BusSelector5/1 -> Ftn_IdControl/5(mCTRL_sIdeRef)  "<mCTRL_sIdeRef>"
  BusSelector5/3 -> Ftn_IdControl/7(mCTRL_sIqe), [mCTRL_sIqe]  "<mCTRL_sIqe>"
  BusSelector5/2 -> Ftn_IdControl/6(mCTRL_sIde), [mCTRL_sIde]  "<mCTRL_sIde>"
  bCurrRefSelOut/1 -> BusSelector5/1
  BusSelector5/4 -> [sTheta]  "<sTheta>"
  BusSelector5/5 -> Ftn_IqControl/1(mCTRL_sIqeRef)  "<mCTRL_sIqeRef>"
  [mCTRL_sIqe] -> Ftn_IqControl/2(mCTRL_sIqe)
  [mCTRL_sIde] -> Ftn_IqControl/3(mCTRL_sIde)
  BusSelector2/4 -> [mMCVG_sCurrKiq]  "<mMCVG_sCCG_Kiq>"
  BusSelector2/2 -> [mMCVG_sCurrKpq]  "<mMCVG_sCCG_Kpq>"

== system e03_MtrCtrl_MtrCtrl/Nftn_MotorControl/Ftn_MtrMdeComn/Nftn_GenBusFromMerOut ==
  note: Input:
      | Description:
      | Output:
  aMerOutCCurrTheta : Inport
  BusCreator1 : BusCreator  Inputs=4
  Demux1 : Demux
  SignalConversion{,1..3} (4 alike) : SignalConversion  OverrideOpt=off
  mCTRL_sIsRef : Outport  Description=■ 설명: 전류 지령  OutMin=-49.498  OutMax=49.498
      settings: AttributesFormatString=%<Description>
  bMerOutCurrTheta : Outport  Description=|  Port=2
      | ■ 설명: 제어 모드 전류 출력 Mux 신호
      | -.[0] : 전압/전류/토크 지령
      | -.[1] : d축 전류
      | -.[2] : q축 전류
      | -.[3] : 추정 위치
      settings: AttributesFormatString=%<Description>
  wires:
  Demux1/4 -> SignalConversion3/1  "MuxOut_sAppTheta"
  Demux1/1 -> SignalConversion/1  "MuxOut_sIsRef"
  Demux1/3 -> SignalConversion2/1  "MuxOut_sIqe"
  aMerOutCCurrTheta/1 -> Demux1/1
  BusCreator1/1 -> bMerOutCurrTheta/1  "bMerOutCurrTheta"
  Demux1/2 -> SignalConversion1/1  "MuxOut_sIde"
  SignalConversion/1 -> BusCreator1/1, mCTRL_sIsRef/1  "mCTRL_sIsRef"
  SignalConversion1/1 -> BusCreator1/2  "sIde"
  SignalConversion2/1 -> BusCreator1/3  "sIqe"
  SignalConversion3/1 -> BusCreator1/4  "sAppTheta"

== system e03_MtrCtrl_MtrCtrl/Nftn_MotorControl/Ftn_MtrMdeComn/Nftn_MtrMdeCmSpdCm ==
  note: Input:
      | Description:
      | Output:
  note: [TQ8, SPD16, PST32]
  bSCHED : Inport
  bCRX : Inport  Port=2
  bMCEST : Inport  Port=3
  bSMDE : Inport  Port=4
  bBSWGVAL : Inport  Port=5
  bMCVG : Inport  Port=6
  uAppCtrlMde : Inport  Port=7
  ActionPort : ActionPort  ActionPortLabel=case [ 8 16 32 ]:
  BusSelector : BusSelector  OutputSignals=mCRX_sVltCurrTqCmd
  BusSelector1 : BusSelector  OutputSignals=mBSW_sTime,mBSW_sOutloopTime,mBSW_sTimePstCtrl,mBSW_sInvTimePstCtrl
  BusSelector2 : BusSelector  OutputSignals=mSched_i32CntForSch,mSched_uFlagSpdCtrl,mSched_uFlagSpdSlop
  BusSelector3 : BusSelector  OutputSignals=mMCVG_sTqSlpRising,mMCVG_sTqSlpFalling,mMCVG_sSpdSlpRising,mMCVG_sSpdSlpFalling,mMCVG_sSCG_Kp,mMCVG_sSCG_Ki,mMCVG_sSCG_Ka,mMCVG_sPCG_Kp,mMCVG_sPCG_Ki,mMCVG_sPCG_Kd,mMCVG_sPCG_Ka,mMCVG_sPCG_Apst
  BusSelector4 : BusSelector  OutputSignals=mSMDE_sSpdRef,mSMDE_sSpdRefInSeqOut,mSMDE_i64PstRef,mSMDE_sSpdLimit
  BusSelector5 : BusSelector  OutputSignals=mMTPST_i64TurretPst,mMTPST_sWm
  Ftn_TqSpdPstCtrl : Subsystem  TreatAsAtomicUnit=on
      settings: RTWSystemCode=Nonreusable function  RTWFcnNameOpts=Use subsystem name
  sIsRefIdqeTheta5 : Outport  Description=|  VectorParamsAs1DForOutWhenUnconnected=off
      | ■ 설명: 제어 모드 전류 출력 Mux 신호
      | -.[0] : 전압/전류/토크 지령
      | -.[1] : d축 전류
      | -.[2] : q축 전류
      | -.[3] : 추정 위치
      settings: AttributesFormatString=|
      | ■ SWC Name: %<Parent>
      | ■ DataType: single
      | ■ Max: %<OutMax>
      | ■ Min: %<OutMin>
      | %<Description>
  mCTRL_sSpdRefIn : Outport  Description=■ 설명: Speed Reference  Port=2  VectorParamsAs1DForOutWhenUnconnected=off
      settings: AttributesFormatString=|
      | ■ SWC Name: %<Parent>
      | ■ DataType: single
      | ■ Max: %<OutMax>
      | ■ Min: %<OutMin>
      | %<Description>
  mCTRL_sTqRefIn : Outport  Description=■ 설명: Tq Slop Reference  Port=3  VectorParamsAs1DForOutWhenUnconnected=off
      settings: AttributesFormatString=|
      | ■ SWC Name: %<Parent>
      | ■ DataType: single
      | ■ Max: %<OutMax>
      | ■ Min: %<OutMin>
      | %<Description>
  wires:
  Ftn_TqSpdPstCtrl/2(mCTRL_sTqRefIn) -> mCTRL_sTqRefIn/1
  uAppCtrlMde/1 -> Ftn_TqSpdPstCtrl/1(uAppCtrlMde)
  Ftn_TqSpdPstCtrl/3(mCTRL_sSpdRefIn) -> mCTRL_sSpdRefIn/1
  Ftn_TqSpdPstCtrl/1(sIsRefIdqeTheta5) -> sIsRefIdqeTheta5/1
  bBSWGVAL/1 -> BusSelector1/1
  BusSelector1/2 -> Ftn_TqSpdPstCtrl/4(mBSW_sOutloopTime)  "<mBSW_sOutloopTime>"
  bSMDE/1 -> BusSelector4/1
  BusSelector4/1 -> Ftn_TqSpdPstCtrl/7(mSMDE_sSpdRef)  "<mSMDE_sSpdRef>"
  BusSelector4/2 -> Ftn_TqSpdPstCtrl/8(mSMDE_sSpdRefInSeqOut)  "<mSMDE_sSpdRefInSeqOut>"
  BusSelector/1 -> Ftn_TqSpdPstCtrl/2(mCRX_sVltCurrTqCmd)  "<mCRX_sVltCurrTqCmd>"
  bCRX/1 -> BusSelector/1
  bMCVG/1 -> BusSelector3/1
  BusSelector3/3 -> Ftn_TqSpdPstCtrl/13(mMCVG_sSpdSlopRising)  "<mMCVG_sSpdSlpRising>"
  BusSelector3/4 -> Ftn_TqSpdPstCtrl/14(mMCVG_sSpdSlopFalling)  "<mMCVG_sSpdSlpFalling>"
  BusSelector3/5 -> Ftn_TqSpdPstCtrl/15(mMCVG_sSpdGainKp)  "<mMCVG_sSCG_Kp>"
  BusSelector3/6 -> Ftn_TqSpdPstCtrl/16(mMCVG_sSpdGainKi)  "<mMCVG_sSCG_Ki>"
  BusSelector3/7 -> Ftn_TqSpdPstCtrl/17(mMCVG_sSpdGainKa)  "<mMCVG_sSCG_Ka>"
  BusSelector5/2 -> Ftn_TqSpdPstCtrl/24(mMTPST_sWm)  "<mMTPST_sWm>"
  bMCEST/1 -> Ftn_TqSpdPstCtrl/25(bMCEST), BusSelector5/1
  bSCHED/1 -> BusSelector2/1
  BusSelector2/3 -> Ftn_TqSpdPstCtrl/28(mSched_uFlagSpdSlop)  "<mSched_uFlagSpdSlop>"
  BusSelector2/2 -> Ftn_TqSpdPstCtrl/27(mSched_uFlagSpdCtrl)  "<mSched_uFlagSpdCtrl>"
  BusSelector3/1 -> Ftn_TqSpdPstCtrl/11(mMCVG_sTqSlpRising)  "<mMCVG_sTqSlpRising>"
  BusSelector3/2 -> Ftn_TqSpdPstCtrl/12(mMCVG_sTqSlpFalling)  "<mMCVG_sTqSlpFalling>"
  BusSelector1/1 -> Ftn_TqSpdPstCtrl/3(mBSW_sTime)  "<mBSW_sTime>"
  BusSelector3/8 -> Ftn_TqSpdPstCtrl/18(mMCVG_sPCG_Kp)  "<mMCVG_sPCG_Kp>"
  BusSelector3/9 -> Ftn_TqSpdPstCtrl/19(mMCVG_sPCG_Ki)  "<mMCVG_sPCG_Ki>"
  BusSelector3/10 -> Ftn_TqSpdPstCtrl/20(mMCVG_sPCG_Kd)  "<mMCVG_sPCG_Kd>"
  BusSelector3/11 -> Ftn_TqSpdPstCtrl/21(mMCVG_sPCG_Ka)  "<mMCVG_sPCG_Ka>"
  BusSelector3/12 -> Ftn_TqSpdPstCtrl/22(mMCVG_sPCG_Apst)  "<mMCVG_sPCG_Apst>"
  BusSelector1/3 -> Ftn_TqSpdPstCtrl/5(mBSW_sTimePstCtrl)  "<mBSW_sTimePstCtrl>"
  BusSelector2/1 -> Ftn_TqSpdPstCtrl/26(mSched_i32CntForSch)  "<mSched_i32CntForSch>"
  BusSelector4/3 -> Ftn_TqSpdPstCtrl/9(mSMDE_i64PstRef)  "<mSMDE_i64PstRef>"
  BusSelector5/1 -> Ftn_TqSpdPstCtrl/23(mMTPST_i64TurretPst)  "<mMTPST_i64TurretPst>"
  BusSelector1/4 -> Ftn_TqSpdPstCtrl/6(mBSW_sInvTimePstCtrl)  "<mBSW_sInvTimePstCtrl>"
  BusSelector4/4 -> Ftn_TqSpdPstCtrl/10(mSMDE_sSpdLimit)  "<mSMDE_sSpdLimit>"

== system e03_MtrCtrl_MtrCtrl/Nftn_MotorControl/Ftn_MtrMdeComn/Ftn_CurrRefSelection/Nftn_GenArryOut ==
  note: Input:
      | Description:
      | Output:
  sIdqeRef : Inport
  sIde : Inport  Port=2
  sIqe : Inport  Port=3
  sAppTheta : Inport  Port=4
  BusCreator : BusCreator  Inputs=5
  BusSelector1 : BusSelector  OutputSignals=sIdeRefCurrMde,sIqeRefCurrMde
  SignalConversion{,1..4} (5 alike) : SignalConversion  OverrideOpt=off
  bCurrRefSelOut : Outport
  wires:
  BusSelector1/2 -> SignalConversion1/1  "<sIqeRefCurrMde>"
  BusSelector1/1 -> SignalConversion/1  "<sIdeRefCurrMde>"
  sIdqeRef/1 -> BusSelector1/1
  sIde/1 -> SignalConversion2/1
  sIqe/1 -> SignalConversion3/1
  sAppTheta/1 -> SignalConversion4/1
  BusCreator/1 -> bCurrRefSelOut/1  "bCurrRefSelOut"
  SignalConversion3/1 -> BusCreator/4  "mCTRL_sIqe"
  SignalConversion2/1 -> BusCreator/3  "mCTRL_sIde"
  SignalConversion4/1 -> BusCreator/5  "sTheta"
  SignalConversion1/1 -> BusCreator/2  "mCTRL_sIqeRef"
  SignalConversion/1 -> BusCreator/1  "mCTRL_sIdeRef"

== system e03_MtrCtrl_MtrCtrl/Nftn_MotorControl/Ftn_MtrMdeComn/Ftn_CurrRefSelection/Nftn_SftCurrMde ==
  note: Input:
      | Description:
      | Output:
  uAppCtrlMde : Inport
  mBSW_sTime : Inport  Port=2
  mCRX_sFreqBetaCmd : Inport  Port=3
  mMCVG_sCurrSlopRising : Inport  Port=4
  mMCVG_sCurrSlopFalling : Inport  Port=5
  mCTRL_sIsRef : Inport  Port=6
  Constant : Constant  Value=E03MCMV.uSoftMdeCurr
  Merge : Merge
  Nftn_CalIsBeta2IdqRef : Subsystem
      settings: RTWSystemCode=Nonreusable function  RTWFcnNameOpts=Use subsystem name
  Nftn_GensAppIeRefLim : Subsystem
  Nftn_SftMdeCurrBypass : Subsystem
  Nftn_SftMdeCurrStart : Subsystem
      settings: RTWFcnNameOpts=Use subsystem name
  SwitchCase : SwitchCase  CaseConditions={ 2}
  mCTRL_sIsRefIn : Outport  VectorParamsAs1DForOutWhenUnconnected=off
  sIdqeRef : Outport  Port=2  VectorParamsAs1DForOutWhenUnconnected=off
  wires:
  SwitchCase/1 -> Nftn_SftMdeCurrStart/Action
  Nftn_SftMdeCurrStart/1(sIsRefIn2) -> Merge/2
  SwitchCase/2 -> Nftn_SftMdeCurrBypass/Action
  Nftn_SftMdeCurrBypass/1(sIsRefIn1) -> [sIsRefIn1]
  [sIsRefIn1] -> Merge/1
  Merge/1 -> mCTRL_sIsRefIn/1, Nftn_CalIsBeta2IdqRef/1(mCTRL_sIsRefIn)  "mCTRL_sIsRefIn"
  Nftn_GensAppIeRefLim/1(sIsRefLimed) -> Nftn_SftMdeCurrStart/1(sIsRefLimed), Nftn_SftMdeCurrBypass/1(sIsRefLimed)
  mCTRL_sIsRef/1 -> Nftn_GensAppIeRefLim/1(mCTRL_sIsRef)
  uAppCtrlMde/1 -> Nftn_CalIsBeta2IdqRef/3(uAppCtrlMde)
  Nftn_CalIsBeta2IdqRef/1(sIdqeRef) -> sIdqeRef/1
  mBSW_sTime/1 -> Nftn_SftMdeCurrStart/2(mBSW_sTime)
  mCRX_sFreqBetaCmd/1 -> Nftn_CalIsBeta2IdqRef/2(mCRX_sFreqBetaCmd)
  mMCVG_sCurrSlopRising/1 -> Nftn_SftMdeCurrStart/3(mMCVG_sCurrSlopRising)
  mMCVG_sCurrSlopFalling/1 -> Nftn_SftMdeCurrStart/4(mMCVG_sCurrSlopFalling)
  Constant/1 -> SwitchCase/1  "uSoftMdeCurr"

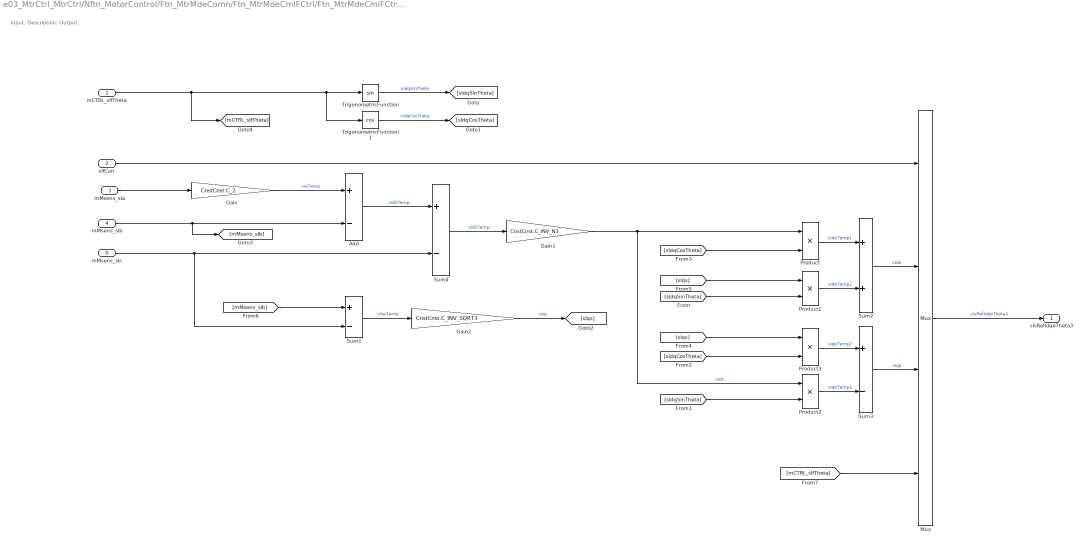
== system e03_MtrCtrl_MtrCtrl/Nftn_MotorControl/Ftn_MtrMdeComn/Ftn_MtrMdeCmIFCtrl/Ftn_MtrMdeCmIFCtrlB ==
  note: Input:
      | Description:
      | Output:
  mCTRL_sIfTheta : Inport  Description=■ 설명: IF - 센서리스 전환시 추정 위치  OutMin=0  OutMax=6.2832
      settings: AttributesFormatString=%<Description>
  sIfCurr : Inport  Description=■ 설명: (IF 제어시) 상전류 지령  Port=2  OutMin=0  OutMax=32.56
      settings: AttributesFormatString=%<Description>
  mMsens_sIa : Inport  Description=■ 설명: 모터 A상 전류  Port=3  OutMin=-162.6  OutMax=162.6
      settings: AttributesFormatString=%<Description>
  mMsens_sIb : Inport  Description=■ 설명: 모터 B상 전류  Port=4  OutMin=-162.6  OutMax=162.6
      settings: AttributesFormatString=%<Description>
  mMsens_sIc : Inport  Description=■ 설명: 모터 C상 전류  Port=5  OutMin=-325.2  OutMax=325.2
      settings: AttributesFormatString=%<Description>
  Add : Sum  Inputs=+-
  Gain : Gain  Gain=CnstCnst.C_2
  Gain1 : Gain  Gain=CnstCnst.C_INV_N3
  Gain2 : Gain  Gain=CnstCnst.C_INV_SQRT3
  Mux : Mux
  Product{,1..3} (4 alike) : Product  RndMeth=Zero
  Sum1 : Sum  Inputs=+-
  Sum2 : Sum
  Sum3 : Sum  Inputs=+-
  Sum4 : Sum  Inputs=+-
  TrigonometricFunction : Trigonometry
  TrigonometricFunction1 : Trigonometry  Operator=cos
  sIsRefIdqeTheta3 : Outport  Description=|  OutMin=-398.3  OutMax=398.3
      | ■ 설명: 제어 모드 전류 출력 Mux 신호
      | -.[0] : 전압/전류/토크 지령
      | -.[1] : d축 전류
      | -.[2] : q축 전류
      | -.[3] : 추정 위치
      settings: AttributesFormatString=%<Description>
  wires:
  sIfCurr/1 -> Mux/1
  Mux/1 -> sIsRefIdqeTheta3/1  "sIsRefIdqeTheta3"
  Product3/1 -> Sum3/1  "sIqeTemp2"
  mCTRL_sIfTheta/1 -> [mCTRL_sIfTheta], TrigonometricFunction/1, TrigonometricFunction1/1
  [sIdqCosTheta] -> Product/2
  [sIqs] -> Product1/1
  Gain2/1 -> [sIqs]  "sIqs"
  [mMsens_sIb] -> Sum1/1
  Product/1 -> Sum2/1  "sIdeTemp1"
  [sIdqSinTheta] -> Product2/2
  Gain1/1 -> Product2/1, Product/1  "sIds"
  [sIdqSinTheta] -> Product1/2
  mMsens_sIb/1 -> [mMsens_sIb], Add/2
  Product2/1 -> Sum3/2  "sIqeTemp1"
  Product1/1 -> Sum2/2  "sIdeTemp2"
  TrigonometricFunction1/1 -> [sIdqCosTheta]  "sIdqCosTheta"
  Sum2/1 -> Mux/2  "sIde"
  [sIqs] -> Product3/1
  Sum3/1 -> Mux/3  "sIqe"
  mMsens_sIa/1 -> Gain/1
  Sum1/1 -> Gain2/1  "sIqsTemp"
  Gain/1 -> Add/1  "sIaTemp"
  Sum4/1 -> Gain1/1  "sIdsTemp"
  TrigonometricFunction/1 -> [sIdqSinTheta]  "sIdqSinTheta"
  mMsens_sIc/1 -> Sum1/2, Sum4/2
  Add/1 -> Sum4/1  "sIdsTemp"
  [sIdqCosTheta] -> Product3/2
  [mCTRL_sIfTheta] -> Mux/4

== system e03_MtrCtrl_MtrCtrl/Nftn_MotorControl/Ftn_MtrMdeComn/Ftn_MtrMdeCmIFCtrl/Nftn_MtrMdeCmIFCtrlA ==
  note: Input:
      | Description:
      | Output:
  mBSW_sTime : Inport  Description=■ 설명: 주기, sTime (1/14kH)  OutMin=0  OutMax=0.0000714286
      settings: AttributesFormatString=%<Description>
  mSMDE_sIfFreqSeqOut : Inport  Description=■ 설명: IF Control Frequency out  Port=2  OutMin=0  OutMax=54
      settings: AttributesFormatString=%<Description>
  CB_C_PI2 : Constant  Value=CnstCnst.C_PI2
  CB_E03MCMV_sIfCurr : Constant  Value=E03MCMV.sIfCurr
  CB_E03MCMV_sIfSetFreq : Constant  Value=E03MCMV.sIfSetFreq
  CB_E03MCMV_sIfTsec : Constant  Value=E03MCMV.sIfTsec
  Chart : Stateflow chart
  UnitDelay : UnitDelay  InitialCondition=E03MCMV.sIfInitTheta  SampleTime=-1  StateName=sIfThetaZ  HasFrameUpgradeWarning=on
      settings: AttributesFormatString=%<InitialCondition>
  mCTRL_sIfFreq : Outport  Description=■ 설명: (IF 제어시) 주파수 지령  OutMin=0  OutMax=54
      settings: AttributesFormatString=%<Description>
  mCTRL_sIfTheta : Outport  Description=■ 설명: (IF 제어시) 추정 위치  Port=2  OutMin=0  OutMax=6.2832
      settings: AttributesFormatString=%<Description>
  sIfCurr : Outport  Description=■ 설명: (IF 제어시) 상전류 지령  Port=3  OutMin=0  OutMax=32.56
      settings: AttributesFormatString=%<Description>
  wires:
  mBSW_sTime/1 -> Chart/1(mBSW_sTime)
  mSMDE_sIfFreqSeqOut/1 -> Chart/2(mSMDE_sIfFreqSeqOut)
  CB_E03MCMV_sIfCurr/1 -> sIfCurr/1  "sIfCurr"
  Chart/1(mCTRL_sIfFreq) -> mCTRL_sIfFreq/1
  UnitDelay/1 -> Chart/6(sIfThetaZ)  "sIfThetaZ"
  Chart/2(mCTRL_sIfTheta) -> mCTRL_sIfTheta/1, UnitDelay/1
  CB_C_PI2/1 -> Chart/5(C_PI2)  "C_PI2"
  CB_E03MCMV_sIfSetFreq/1 -> Chart/3(sIfSetFreq)  "sIfSetFreq"
  CB_E03MCMV_sIfTsec/1 -> Chart/4(sIfTsec)  "sIfTsec"
